simulink model "KamlanMF"  (R2018a)
settings: Solver=ode4  StartTime=0.0  StopTime=50  FixedStep=0.01  RelTol=1e-3
values from neighbouring files (symbols this model uses):
  b = 5    [Kalman.m]    (also in fcn.m; untitled2.m)
  k = 5    [Kalman.m]    (also in fcn.m; temtProp.m = 100; untitled2.m)
  m = 10    [Kalman.m]    (also in fcn.m; temtProp.m; untitled2.m)
  R = 10    [Kalman.m]    (also in fcn.m = 0.0001; temtProp.m = 0.0001; untitled2.m = 1-e4)
  Ts = 0.1    [temtProp.m]    (also in untitled2.m = 0.01)
libraries: simulink x1
settings Model: Creator=Ali  LastModifiedBy=Ali

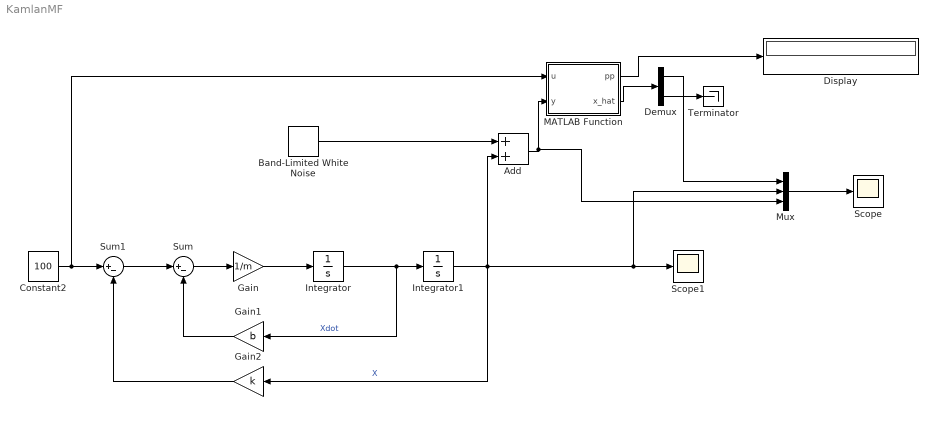
== system KamlanMF ==
  Add : Sum
  Band-Limited White Noise : simulink/Sources/Band-Limited White Noise  Cov=R*Ts  Ts=Ts  seed=[23341]
  Constant2 : Constant  Value=100
  Demux : Demux  Outputs=2
  Display : Display
  Gain : Gain  Gain=1/m
  Gain1 : Gain  Gain=b
  Gain2 : Gain  Gain=k
  Integrator : Integrator
  Integrator1 : Integrator  InitialCondition=0.01
  MATLAB Function : MATLAB Function  TreatAsAtomicUnit=on
  Mux : Mux  Inputs=3
  Scope : Scope
  Scope1 : Scope
  Sum : Sum  Inputs=|+-
  Sum1 : Sum  Inputs=|+-
  Terminator : Terminator
  wires:
  Gain/1 -> Integrator/1
  Constant2/1 -> MATLAB Function/1(u), Sum1/1
  Integrator1/1 -> Add/2, Gain2/1, Mux/2, Scope1/1  "X"
  Gain1/1 -> Sum/2
  Gain2/1 -> Sum1/2
  Sum1/1 -> Sum/1
  Integrator/1 -> Gain1/1, Integrator1/1  "Xdot"
  Sum/1 -> Gain/1
  MATLAB Function/2(x_hat) -> Demux/1
  Demux/2 -> Terminator/1
  Demux/1 -> Mux/1
  Mux/1 -> Scope/1
  Add/1 -> Mux/3, MATLAB Function/2(y)
  Band-Limited White Noise/1 -> Add/1
  MATLAB Function/1(pp) -> Display/1

== matlab function KamlanMF/MATLAB Function ==
  settings: updateMethod=DISCRETE
  data: pp output; u input; x_hat output; y input
function [pp,x_hat]= fcn(u, y)
pp = zeros(2);
x_hat = zeros(2,1);
m = 10;
b = 5;
k = 5;
A = [0 1;...
    -k/m -b/m];
B = [0; 1/m];
C = [0 1];
R = 1e-4;
Q = 1e-4;
x_zero = [0; 0];
x_hzero = [10; 0];
     persistent p_pri p K xhat
     if isempty(xhat)
         xhat = x_hzero;
         return
     end
     if isempty(p)
         p = diag([0 20]);
         return
     end
x_pri = A*xhat+B*u;
p_pri = A*p*A + Q;
K = (p_pri*C')/(C*p_pri*C'+R);
xhat = x_pri + K*(y-C*x_pri);
p = (eye(2)-K*C)*p_pri;
x_hat = xhat;
pp = p;
